simulink model "SIMULINK_PID_Tracking_R18b"  (R2018b)
settings: Solver=FixedStepAuto  StartTime=0.0  StopTime=sim_end_time  FixedStep=fixed_step_size  RelTol=1e-3
undefined symbols (not defined in the file): a, act_end, b, battery_threshold, bb, draw_gif, droneyeeUAV2_NUM, droneyeeUAV3_NUM, droneyeeUAV4_NUM, droneyeeUAV5_NUM, fixed_step_size, k, KD_x, KD_y, kd_z, KDD_x, KDD_y, KI_x, KI_y, ki_z, KII_x, KII_y, KP_x, KP_y, kp_z, KPP_x, KPP_y, lmt, omega, R, sim_end_time, uav10num, uav1num, uav2num, uav3num, uav4num, uav5num, uav6num, uav7num, uav8num, uav9num, UAV_NUM, Vel_Switch_1, Vel_Switch_10, Vel_Switch_11, Vel_Switch_12, Vel_Switch_13, Vel_Switch_14, Vel_Switch_15, Vel_Switch_16, Vel_Switch_17, Vel_Switch_18, Vel_Switch_19, Vel_Switch_2, Vel_Switch_20, Vel_Switch_3, Vel_Switch_4, Vel_Switch_5, Vel_Switch_6, Vel_Switch_7 ... (+12)
libraries: simulink x120, aerolibanimutils x1
(part 9 of 10)

== system SIMULINK_PID_Tracking_R18b/send_ctrl_signal_car1/Send Command 4/Subsystem ==
  In1 : Inport
  Compare To Constant2 : simulink/Logic and Bit Operations/Compare To Constant  relop=~=  const=0  OutDataTypeStr=boolean
  Demux : Demux  Outputs=2
  Logical Operator1 : Logic  Operator=OR  AllPortsSameDT=off  OutDataTypeStr=boolean
  Out1 : Outport
  wires:
  Demux/2 -> Logical Operator1/2
  Logical Operator1/1 -> Out1/1
  Demux/1 -> Logical Operator1/1
  Compare To Constant2/1 -> Demux/1
  In1/1 -> Compare To Constant2/1

== system SIMULINK_PID_Tracking_R18b/send_ctrl_signal_car1/Send Command 5/Subsystem ==
  In1 : Inport
  Compare To Constant2 : simulink/Logic and Bit Operations/Compare To Constant  relop=~=  const=0  OutDataTypeStr=boolean
  Demux : Demux  Outputs=2
  Logical Operator1 : Logic  Operator=OR  AllPortsSameDT=off  OutDataTypeStr=boolean
  Out1 : Outport
  wires:
  Demux/2 -> Logical Operator1/2
  Logical Operator1/1 -> Out1/1
  Demux/1 -> Logical Operator1/1
  Compare To Constant2/1 -> Demux/1
  In1/1 -> Compare To Constant2/1

== system SIMULINK_PID_Tracking_R18b/send_ctrl_signal_car1/Send Command 6/Subsystem ==
  In1 : Inport
  Compare To Constant2 : simulink/Logic and Bit Operations/Compare To Constant  relop=~=  const=0  OutDataTypeStr=boolean
  Demux : Demux  Outputs=2
  Logical Operator1 : Logic  Operator=OR  AllPortsSameDT=off  OutDataTypeStr=boolean
  Out1 : Outport
  wires:
  Demux/2 -> Logical Operator1/2
  Logical Operator1/1 -> Out1/1
  Demux/1 -> Logical Operator1/1
  Compare To Constant2/1 -> Demux/1
  In1/1 -> Compare To Constant2/1

== system SIMULINK_PID_Tracking_R18b/send_ctrl_signal_car1/Send Command 7/Subsystem ==
  In1 : Inport
  Compare To Constant2 : simulink/Logic and Bit Operations/Compare To Constant  relop=~=  const=0  OutDataTypeStr=boolean
  Demux : Demux  Outputs=2
  Logical Operator1 : Logic  Operator=OR  AllPortsSameDT=off  OutDataTypeStr=boolean
  Out1 : Outport
  wires:
  Demux/2 -> Logical Operator1/2
  Logical Operator1/1 -> Out1/1
  Demux/1 -> Logical Operator1/1
  Compare To Constant2/1 -> Demux/1
  In1/1 -> Compare To Constant2/1

== system SIMULINK_PID_Tracking_R18b/send_ctrl_signal_car1/Send Command 8/Subsystem ==
  In1 : Inport
  Compare To Constant2 : simulink/Logic and Bit Operations/Compare To Constant  relop=~=  const=0  OutDataTypeStr=boolean
  Demux : Demux  Outputs=2
  Logical Operator1 : Logic  Operator=OR  AllPortsSameDT=off  OutDataTypeStr=boolean
  Out1 : Outport
  wires:
  Demux/2 -> Logical Operator1/2
  Logical Operator1/1 -> Out1/1
  Demux/1 -> Logical Operator1/1
  Compare To Constant2/1 -> Demux/1
  In1/1 -> Compare To Constant2/1

== system SIMULINK_PID_Tracking_R18b/send_ctrl_signal_car1/Send Command 9/Subsystem ==
  In1 : Inport
  Compare To Constant2 : simulink/Logic and Bit Operations/Compare To Constant  relop=~=  const=0  OutDataTypeStr=boolean
  Demux : Demux  Outputs=2
  Logical Operator1 : Logic  Operator=OR  AllPortsSameDT=off  OutDataTypeStr=boolean
  Out1 : Outport
  wires:
  Demux/2 -> Logical Operator1/2
  Logical Operator1/1 -> Out1/1
  Demux/1 -> Logical Operator1/1
  Compare To Constant2/1 -> Demux/1
  In1/1 -> Compare To Constant2/1

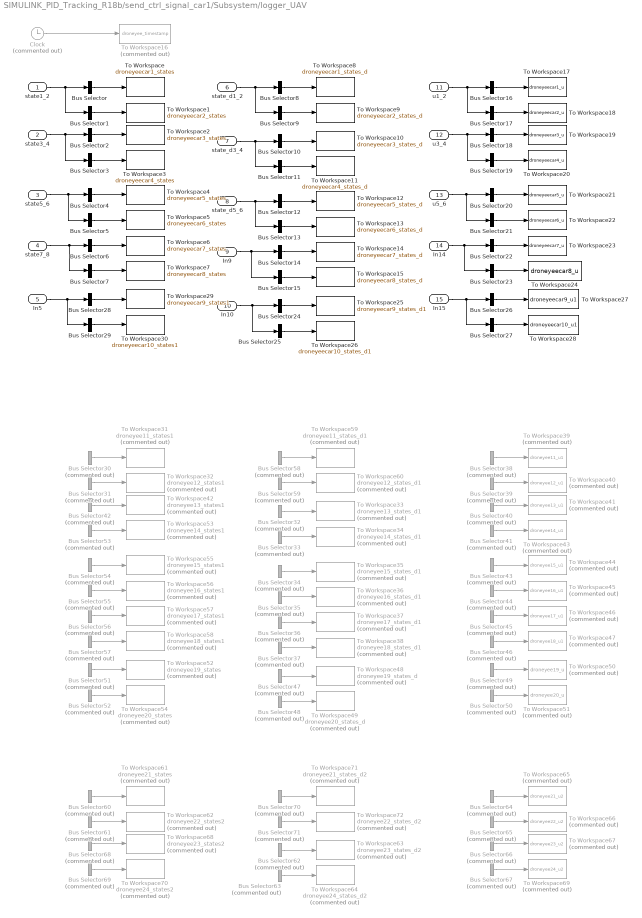
== system SIMULINK_PID_Tracking_R18b/send_ctrl_signal_car1/Subsystem/logger_UAV ==
  state1_2 : Inport
  state3_4 : Inport  Port=2
  state5_6 : Inport  Port=3
  state7_8 : Inport  Port=4
  In5 : Inport  Port=5
  state_d1_2 : Inport  Port=6
  state_d3_4 : Inport  Port=7
  state_d5_6 : Inport  Port=8
  In9 : Inport  Port=9
  In10 : Inport  Port=10
  u1_2 : Inport  Port=11
  u3_4 : Inport  Port=12
  u5_6 : Inport  Port=13
  In14 : Inport  Port=14
  In15 : Inport  Port=15
  Bus Selector : BusSelector  OutputSignals=droneyeeCAR1_states  OutputAsBus=on
  Bus Selector1 : BusSelector  OutputSignals=droneyeeCAR2_states  OutputAsBus=on
  Bus Selector10 : BusSelector  OutputSignals=droneyeeCAR3_d  OutputAsBus=on
  Bus Selector11 : BusSelector  OutputSignals=droneyeeCAR4_d  OutputAsBus=on
  Bus Selector12 : BusSelector  OutputSignals=droneyeeCAR5_d  OutputAsBus=on
  Bus Selector13 : BusSelector  OutputSignals=droneyeeCAR6_d  OutputAsBus=on
  Bus Selector14 : BusSelector  OutputSignals=droneyeeCAR7_d  OutputAsBus=on
  Bus Selector15 : BusSelector  OutputSignals=droneyeeCAR8_d  OutputAsBus=on
  Bus Selector16 : BusSelector  OutputSignals=CAR1.u_vx,CAR1.u_vy,CAR1.u_vz,CAR1.u_rate_roll,CAR1.u_rate_pitch,CAR1.u_rate_yaw  OutputAsBus=on
  Bus Selector17 : BusSelector  OutputSignals=CAR2.u_vx,CAR2.u_vy,CAR2.u_vz,CAR2.u_rate_roll,CAR2.u_rate_pitch,CAR2.u_rate_yaw  OutputAsBus=on
  Bus Selector18 : BusSelector  OutputSignals=CAR3.u_vx,CAR3.u_vy,CAR3.u_vz,CAR3.u_rate_roll,CAR3.u_rate_pitch,CAR3.u_rate_yaw  OutputAsBus=on
  Bus Selector19 : BusSelector  OutputSignals=CAR4.u_vx,CAR4.u_vy,CAR4.u_vz,CAR4.u_rate_roll,CAR4.u_rate_pitch,CAR4.u_rate_yaw  OutputAsBus=on
  Bus Selector2 : BusSelector  OutputSignals=droneyeeCAR3_states  OutputAsBus=on
  Bus Selector20 : BusSelector  OutputSignals=CAR5  OutputAsBus=on
  Bus Selector21 : BusSelector  OutputSignals=CAR6  OutputAsBus=on
  Bus Selector22 : BusSelector  OutputSignals=CAR7  OutputAsBus=on
  Bus Selector23 : BusSelector  OutputSignals=CAR8  OutputAsBus=on
  Bus Selector24 : BusSelector  OutputSignals=droneyeeCAR9_d  OutputAsBus=on
  Bus Selector25 : BusSelector  OutputSignals=droneyeeCAR10_d  OutputAsBus=on
  Bus Selector26 : BusSelector  OutputSignals=CAR9  OutputAsBus=on
  Bus Selector27 : BusSelector  OutputSignals=CAR10  OutputAsBus=on
  Bus Selector28 : BusSelector  OutputSignals=droneyeeCAR9_states  OutputAsBus=on
  Bus Selector29 : BusSelector  OutputSignals=droneyeeCAR10_states  OutputAsBus=on
  Bus Selector3 : BusSelector  OutputSignals=droneyeeCAR4_states  OutputAsBus=on
  Bus Selector30 : BusSelector  Commented=on  OutputSignals=droneyeeUAV11_states.x1,droneyeeUAV11_states.y1,droneyeeUAV11_states.z1,droneyeeUAV11_states.yaw1,droneyeeUAV11_states.vx1,droneyeeUAV11_states.vy1,droneyeeUAV11_states.vz1  OutputAsBus=on
  Bus Selector31 : BusSelector  Commented=on  OutputSignals=droneyeeUAV12_states.x2,droneyeeUAV12_states.y2,droneyeeUAV12_states.z2,droneyeeUAV12_states.yaw2,droneyeeUAV12_states.vx2,droneyeeUAV12_states.vy2,droneyeeUAV12_states.vz2  OutputAsBus=on
  Bus Selector32 : BusSelector  Commented=on  OutputSignals=droneyeeUAV13_d.x13_d,droneyeeUAV13_d.y13_d,droneyeeUAV13_d.z13_d,droneyeeUAV13_d.yaw13_d  OutputAsBus=on
  Bus Selector33 : BusSelector  Commented=on  OutputSignals=droneyeeUAV14_d.x14_d,droneyeeUAV14_d.y14_d,droneyeeUAV14_d.z14_d,droneyeeUAV14_d.yaw14_d  OutputAsBus=on
  Bus Selector34 : BusSelector  Commented=on  OutputSignals=droneyeeUAV15_d.x15_d,droneyeeUAV15_d.y15_d,droneyeeUAV15_d.z15_d,droneyeeUAV15_d.yaw15_d  OutputAsBus=on
  Bus Selector35 : BusSelector  Commented=on  OutputSignals=droneyeeUAV16_d.x16_d,droneyeeUAV16_d.y16_d,droneyeeUAV16_d.z16_d,droneyeeUAV16_d.yaw16_d  OutputAsBus=on
  Bus Selector36 : BusSelector  Commented=on  OutputSignals=droneyeeUAV17_d.x17_d,droneyeeUAV17_d.y17_d,droneyeeUAV17_d.z17_d,droneyeeUAV17_d.yaw17_d  OutputAsBus=on
  Bus Selector37 : BusSelector  Commented=on  OutputSignals=droneyeeUAV18_d.x18_d,droneyeeUAV18_d.y18_d,droneyeeUAV18_d.z18_d,droneyeeUAV18_d.yaw18_d  OutputAsBus=on
  Bus Selector38 : BusSelector  Commented=on  OutputSignals=uav1.u_vx,uav1.u_vy,uav1.u_vz,uav1.u_rate_roll,uav1.u_rate_pitch,uav1.u_rate_yaw  OutputAsBus=on
  Bus Selector39 : BusSelector  Commented=on  OutputSignals=uav2.u_vx,uav2.u_vy,uav2.u_vz,uav2.u_rate_roll,uav2.u_rate_pitch,uav2.u_rate_yaw  OutputAsBus=on
  Bus Selector4 : BusSelector  OutputSignals=droneyeeCAR5_states  OutputAsBus=on
  Bus Selector40 : BusSelector  Commented=on  OutputSignals=uav3.u_vx,uav3.u_vy,uav3.u_vz,uav3.u_rate_roll,uav3.u_rate_pitch,uav3.u_rate_yaw  OutputAsBus=on
  Bus Selector41 : BusSelector  Commented=on  OutputSignals=uav4.u_vx,uav4.u_vy,uav4.u_vz,uav4.u_rate_roll,uav4.u_rate_pitch,uav4.u_rate_yaw  OutputAsBus=on
  Bus Selector42 : BusSelector  Commented=on  OutputSignals=droneyeeUAV13_states.x3,droneyeeUAV13_states.y3,droneyeeUAV13_states.z3,droneyeeUAV13_states.yaw3,droneyeeUAV13_states.vx3,droneyeeUAV13_states.vy3,droneyeeUAV13_states.vz3  OutputAsBus=on
  Bus Selector43 : BusSelector  Commented=on  OutputSignals=uav5.u_vx,uav5.u_vy,uav5.u_vz,uav5.u_rate_roll,uav5.u_rate_pitch,uav5.u_rate_yaw  OutputAsBus=on
  Bus Selector44 : BusSelector  Commented=on  OutputSignals=uav6.u_vx,uav6.u_vy,uav6.u_vz,uav6.u_rate_roll,uav6.u_rate_pitch,uav6.u_rate_yaw  OutputAsBus=on
  Bus Selector45 : BusSelector  Commented=on  OutputSignals=uav7.u_vx,uav7.u_vy,uav7.u_vz,uav7.u_rate_roll,uav7.u_rate_pitch,uav7.u_rate_yaw  OutputAsBus=on
  Bus Selector46 : BusSelector  Commented=on  OutputSignals=uav8.u_vx,uav8.u_vy,uav8.u_vz,uav8.u_rate_roll,uav8.u_rate_pitch,uav8.u_rate_yaw  OutputAsBus=on
  Bus Selector47 : BusSelector  Commented=on  OutputSignals=droneyeeUAV19_d.x19_d,droneyeeUAV19_d.y19_d,droneyeeUAV19_d.z19_d,droneyeeUAV19_d.yaw19_d  OutputAsBus=on
  Bus Selector48 : BusSelector  Commented=on  OutputSignals=droneyeeUAV20_d.x20_d,droneyeeUAV20_d.y20_d,droneyeeUAV20_d.z20_d,droneyeeUAV20_d.yaw20_d  OutputAsBus=on
  Bus Selector49 : BusSelector  Commented=on  OutputSignals=uav9.u_vx,uav9.u_vy,uav9.u_vz,uav9.u_rate_roll,uav9.u_rate_pitch,uav9.u_rate_yaw  OutputAsBus=on
  Bus Selector5 : BusSelector  OutputSignals=droneyeeCAR6_states  OutputAsBus=on
  Bus Selector50 : BusSelector  Commented=on  OutputSignals=uav10.u_vx,uav10.u_vy,uav10.u_vz,uav10.u_rate_roll,uav10.u_rate_pitch,uav10.u_rate_yaw  OutputAsBus=on
  Bus Selector51 : BusSelector  Commented=on  OutputSignals=droneyeeUAV19_states.x9,droneyeeUAV19_states.y9,droneyeeUAV19_states.z9,droneyeeUAV19_states.yaw9,droneyeeUAV19_states.vx9,droneyeeUAV19_states.vy9,droneyeeUAV19_states.vz9  OutputAsBus=on
  Bus Selector52 : BusSelector  Commented=on  OutputSignals=droneyeeUAV20_states.x10,droneyeeUAV20_states.y10,droneyeeUAV20_states.z10,droneyeeUAV20_states.yaw10,droneyeeUAV20_states.vx10,droneyeeUAV20_states.vy10,droneyeeUAV20_states.vz10  OutputAsBus=on
  Bus Selector53 : BusSelector  Commented=on  OutputSignals=droneyeeUAV14_states.x4,droneyeeUAV14_states.y4,droneyeeUAV14_states.z4,droneyeeUAV14_states.yaw4,droneyeeUAV14_states.vx4,droneyeeUAV14_states.vy4,droneyeeUAV14_states.vz4  OutputAsBus=on
  Bus Selector54 : BusSelector  Commented=on  OutputSignals=droneyeeUAV15_states.x5,droneyeeUAV15_states.y5,droneyeeUAV15_states.z5,droneyeeUAV15_states.yaw5,droneyeeUAV15_states.vx5,droneyeeUAV15_states.vy5,droneyeeUAV15_states.vz5  OutputAsBus=on
  Bus Selector55 : BusSelector  Commented=on  OutputSignals=droneyeeUAV16_states.x6,droneyeeUAV16_states.y6,droneyeeUAV16_states.z6,droneyeeUAV16_states.yaw6,droneyeeUAV16_states.vx6,droneyeeUAV16_states.vy6,droneyeeUAV16_states.vz6  OutputAsBus=on
  Bus Selector56 : BusSelector  Commented=on  OutputSignals=droneyeeUAV17_states.x7,droneyeeUAV17_states.y7,droneyeeUAV17_states.z7,droneyeeUAV17_states.yaw7,droneyeeUAV17_states.vx7,droneyeeUAV17_states.vy7,droneyeeUAV17_states.vz7  OutputAsBus=on
  Bus Selector57 : BusSelector  Commented=on  OutputSignals=droneyeeUAV18_states.x8,droneyeeUAV18_states.y8,droneyeeUAV18_states.z8,droneyeeUAV18_states.yaw8,droneyeeUAV18_states.vx8,droneyeeUAV18_states.vy8,droneyeeUAV18_states.vz8  OutputAsBus=on
  Bus Selector58 : BusSelector  Commented=on  OutputSignals=droneyeeUAV11_d.x11_d,droneyeeUAV11_d.y11_d,droneyeeUAV11_d.z11_d,droneyeeUAV11_d.yaw11_d  OutputAsBus=on
  Bus Selector59 : BusSelector  Commented=on  OutputSignals=droneyeeUAV12_d.x12_d,droneyeeUAV12_d.y12_d,droneyeeUAV12_d.z12_d,droneyeeUAV12_d.yaw12_d  OutputAsBus=on
  Bus Selector6 : BusSelector  OutputSignals=droneyeeCAR7_states  OutputAsBus=on
  Bus Selector60 : BusSelector  Commented=on  OutputSignals=droneyeeUAV21_states.x1,droneyeeUAV21_states.y1,droneyeeUAV21_states.z1,droneyeeUAV21_states.yaw1,droneyeeUAV21_states.vx1,droneyeeUAV21_states.vy1,droneyeeUAV21_states.vz1  OutputAsBus=on
  Bus Selector61 : BusSelector  Commented=on  OutputSignals=droneyeeUAV22_states.x2,droneyeeUAV22_states.y2,droneyeeUAV22_states.z2,droneyeeUAV22_states.yaw2,droneyeeUAV22_states.vx2,droneyeeUAV22_states.vy2,droneyeeUAV22_states.vz2  OutputAsBus=on
  Bus Selector62 : BusSelector  Commented=on  OutputSignals=droneyeeUAV23_d.x23_d,droneyeeUAV23_d.y23_d,droneyeeUAV23_d.z23_d,droneyeeUAV23_d.yaw23_d  OutputAsBus=on
  Bus Selector63 : BusSelector  Commented=on  OutputSignals=droneyeeUAV24_d.x24_d,droneyeeUAV24_d.y24_d,droneyeeUAV24_d.z24_d,droneyeeUAV24_d.yaw24_d  OutputAsBus=on
  Bus Selector64 : BusSelector  Commented=on  OutputSignals=uav1.u_vx,uav1.u_vy,uav1.u_vz,uav1.u_rate_roll,uav1.u_rate_pitch,uav1.u_rate_yaw  OutputAsBus=on
  Bus Selector65 : BusSelector  Commented=on  OutputSignals=uav2.u_vx,uav2.u_vy,uav2.u_vz,uav2.u_rate_roll,uav2.u_rate_pitch,uav2.u_rate_yaw  OutputAsBus=on
  Bus Selector66 : BusSelector  Commented=on  OutputSignals=uav3.u_vx,uav3.u_vy,uav3.u_vz,uav3.u_rate_roll,uav3.u_rate_pitch,uav3.u_rate_yaw  OutputAsBus=on
  Bus Selector67 : BusSelector  Commented=on  OutputSignals=uav4.u_vx,uav4.u_vy,uav4.u_vz,uav4.u_rate_roll,uav4.u_rate_pitch,uav4.u_rate_yaw  OutputAsBus=on
  Bus Selector68 : BusSelector  Commented=on  OutputSignals=droneyeeUAV23_states.x3,droneyeeUAV23_states.y3,droneyeeUAV23_states.z3,droneyeeUAV23_states.yaw3,droneyeeUAV23_states.vx3,droneyeeUAV23_states.vy3,droneyeeUAV23_states.vz3  OutputAsBus=on
  Bus Selector69 : BusSelector  Commented=on  OutputSignals=droneyeeUAV24_states.x4,droneyeeUAV24_states.y4,droneyeeUAV24_states.z4,droneyeeUAV24_states.yaw4,droneyeeUAV24_states.vx4,droneyeeUAV24_states.vy4,droneyeeUAV24_states.vz4  OutputAsBus=on
  Bus Selector7 : BusSelector  OutputSignals=droneyeeCAR8_states  OutputAsBus=on
  Bus Selector70 : BusSelector  Commented=on  OutputSignals=droneyeeUAV21_d.x21_d,droneyeeUAV21_d.y21_d,droneyeeUAV21_d.z21_d,droneyeeUAV21_d.yaw21_d  OutputAsBus=on
  Bus Selector71 : BusSelector  Commented=on  OutputSignals=droneyeeUAV22_d.x22_d,droneyeeUAV22_d.y22_d,droneyeeUAV22_d.z22_d,droneyeeUAV22_d.yaw22_d  OutputAsBus=on
  Bus Selector8 : BusSelector  OutputSignals=droneyeeCAR1_d  OutputAsBus=on
  Bus Selector9 : BusSelector  OutputSignals=droneyeeCAR2_d  OutputAsBus=on
  Clock : Clock  Commented=on
  To Workspace : ToWorkspace  VariableName=droneyeecar1_states  SampleTime=-1
  To Workspace1 : ToWorkspace  VariableName=droneyeecar2_states  SampleTime=-1
  To Workspace10 : ToWorkspace  VariableName=droneyeecar3_states_d  SampleTime=-1
  To Workspace11 : ToWorkspace  VariableName=droneyeecar4_states_d  SampleTime=-1
  To Workspace12 : ToWorkspace  VariableName=droneyeecar5_states_d  SampleTime=-1
  To Workspace13 : ToWorkspace  VariableName=droneyeecar6_states_d  SampleTime=-1
  To Workspace14 : ToWorkspace  VariableName=droneyeecar7_states_d  SampleTime=-1
  To Workspace15 : ToWorkspace  VariableName=droneyeecar8_states_d  SampleTime=-1
  To Workspace16 : ToWorkspace  Commented=on  VariableName=droneyee_timestamp  SampleTime=-1
  To Workspace17 : ToWorkspace  VariableName=droneyeecar1_u  SampleTime=-1
  To Workspace18 : ToWorkspace  VariableName=droneyeecar2_u  SampleTime=-1
  To Workspace19 : ToWorkspace  VariableName=droneyeecar3_u  SampleTime=-1
  To Workspace2 : ToWorkspace  VariableName=droneyeecar3_states  SampleTime=-1
  To Workspace20 : ToWorkspace  VariableName=droneyeecar4_u  SampleTime=-1
  To Workspace21 : ToWorkspace  VariableName=droneyeecar5_u  SampleTime=-1
  To Workspace22 : ToWorkspace  VariableName=droneyeecar6_u  SampleTime=-1
  To Workspace23 : ToWorkspace  VariableName=droneyeecar7_u  SampleTime=-1
  To Workspace24 : ToWorkspace  VariableName=droneyeecar8_u  SampleTime=-1
  To Workspace25 : ToWorkspace  VariableName=droneyeecar9_states_d1  SampleTime=-1
  To Workspace26 : ToWorkspace  VariableName=droneyeecar10_states_d1  SampleTime=-1
  To Workspace27 : ToWorkspace  VariableName=droneyeecar9_u1  SampleTime=-1
  To Workspace28 : ToWorkspace  VariableName=droneyeecar10_u1  SampleTime=-1
  To Workspace29 : ToWorkspace  VariableName=droneyeecar9_states1  SampleTime=-1
  To Workspace3 : ToWorkspace  VariableName=droneyeecar4_states  SampleTime=-1
  To Workspace30 : ToWorkspace  VariableName=droneyeecar10_states1  SampleTime=-1
  To Workspace31 : ToWorkspace  Commented=on  VariableName=droneyee11_states1  SampleTime=-1
  To Workspace32 : ToWorkspace  Commented=on  VariableName=droneyee12_states1  SampleTime=-1
  To Workspace33 : ToWorkspace  Commented=on  VariableName=droneyee13_states_d1  SampleTime=-1
  To Workspace34 : ToWorkspace  Commented=on  VariableName=droneyee14_states_d1  SampleTime=-1
  To Workspace35 : ToWorkspace  Commented=on  VariableName=droneyee15_states_d1  SampleTime=-1
  To Workspace36 : ToWorkspace  Commented=on  VariableName=droneyee16_states_d1  SampleTime=-1
  To Workspace37 : ToWorkspace  Commented=on  VariableName=droneyee17_states_d1  SampleTime=-1
  To Workspace38 : ToWorkspace  Commented=on  VariableName=droneyee18_states_d1  SampleTime=-1
  To Workspace39 : ToWorkspace  Commented=on  VariableName=droneyee11_u1  SampleTime=-1
  To Workspace4 : ToWorkspace  VariableName=droneyeecar5_states  SampleTime=-1
  To Workspace40 : ToWorkspace  Commented=on  VariableName=droneyee12_u1  SampleTime=-1
  To Workspace41 : ToWorkspace  Commented=on  VariableName=droneyee13_u1  SampleTime=-1
  To Workspace42 : ToWorkspace  Commented=on  VariableName=droneyee13_states1  SampleTime=-1
  To Workspace43 : ToWorkspace  Commented=on  VariableName=droneyee14_u1  SampleTime=-1
  To Workspace44 : ToWorkspace  Commented=on  VariableName=droneyee15_u1  SampleTime=-1
  To Workspace45 : ToWorkspace  Commented=on  VariableName=droneyee16_u1  SampleTime=-1
  To Workspace46 : ToWorkspace  Commented=on  VariableName=droneyee17_u1  SampleTime=-1
  To Workspace47 : ToWorkspace  Commented=on  VariableName=droneyee18_u1  SampleTime=-1
  To Workspace48 : ToWorkspace  Commented=on  VariableName=droneyee19_states_d  SampleTime=-1
  To Workspace49 : ToWorkspace  Commented=on  VariableName=droneyee20_states_d  SampleTime=-1
  To Workspace5 : ToWorkspace  VariableName=droneyeecar6_states  SampleTime=-1
  To Workspace50 : ToWorkspace  Commented=on  VariableName=droneyee19_u  SampleTime=-1
  To Workspace51 : ToWorkspace  Commented=on  VariableName=droneyee20_u  SampleTime=-1
  To Workspace52 : ToWorkspace  Commented=on  VariableName=droneyee19_states  SampleTime=-1
  To Workspace53 : ToWorkspace  Commented=on  VariableName=droneyee14_states1  SampleTime=-1
  To Workspace54 : ToWorkspace  Commented=on  VariableName=droneyee20_states  SampleTime=-1
  To Workspace55 : ToWorkspace  Commented=on  VariableName=droneyee15_states1  SampleTime=-1
  To Workspace56 : ToWorkspace  Commented=on  VariableName=droneyee16_states1  SampleTime=-1
  To Workspace57 : ToWorkspace  Commented=on  VariableName=droneyee17_states1  SampleTime=-1
  To Workspace58 : ToWorkspace  Commented=on  VariableName=droneyee18_states1  SampleTime=-1
  To Workspace59 : ToWorkspace  Commented=on  VariableName=droneyee11_states_d1  SampleTime=-1
  To Workspace6 : ToWorkspace  VariableName=droneyeecar7_states  SampleTime=-1
  To Workspace60 : ToWorkspace  Commented=on  VariableName=droneyee12_states_d1  SampleTime=-1
  To Workspace61 : ToWorkspace  Commented=on  VariableName=droneyee21_states  SampleTime=-1
  To Workspace62 : ToWorkspace  Commented=on  VariableName=droneyee22_states2  SampleTime=-1
  To Workspace63 : ToWorkspace  Commented=on  VariableName=droneyee23_states_d2  SampleTime=-1
  To Workspace64 : ToWorkspace  Commented=on  VariableName=droneyee24_states_d2  SampleTime=-1
  To Workspace65 : ToWorkspace  Commented=on  VariableName=droneyee21_u2  SampleTime=-1
  To Workspace66 : ToWorkspace  Commented=on  VariableName=droneyee22_u2  SampleTime=-1
  To Workspace67 : ToWorkspace  Commented=on  VariableName=droneyee23_u2  SampleTime=-1
  To Workspace68 : ToWorkspace  Commented=on  VariableName=droneyee23_states2  SampleTime=-1
  To Workspace69 : ToWorkspace  Commented=on  VariableName=droneyee24_u2  SampleTime=-1
  To Workspace7 : ToWorkspace  VariableName=droneyeecar8_states  SampleTime=-1
  To Workspace70 : ToWorkspace  Commented=on  VariableName=droneyee24_states2  SampleTime=-1
  To Workspace71 : ToWorkspace  Commented=on  VariableName=droneyee21_states_d2  SampleTime=-1
  To Workspace72 : ToWorkspace  Commented=on  VariableName=droneyee22_states_d2  SampleTime=-1
  To Workspace8 : ToWorkspace  VariableName=droneyeecar1_states_d  SampleTime=-1
  To Workspace9 : ToWorkspace  VariableName=droneyeecar2_states_d  SampleTime=-1
  wires:
  state1_2/1 -> Bus Selector1/1, Bus Selector/1
  Bus Selector/1 -> To Workspace/1
  Bus Selector1/1 -> To Workspace1/1
  Bus Selector3/1 -> To Workspace3/1
  Bus Selector2/1 -> To Workspace2/1
  state3_4/1 -> Bus Selector3/1, Bus Selector2/1
  Bus Selector5/1 -> To Workspace5/1
  Bus Selector4/1 -> To Workspace4/1
  Bus Selector7/1 -> To Workspace7/1
  Bus Selector6/1 -> To Workspace6/1
  Bus Selector9/1 -> To Workspace9/1
  Bus Selector8/1 -> To Workspace8/1
  state_d1_2/1 -> Bus Selector9/1, Bus Selector8/1
  Bus Selector10/1 -> To Workspace10/1
  Bus Selector11/1 -> To Workspace11/1
  Bus Selector12/1 -> To Workspace12/1
  state_d3_4/1 -> Bus Selector11/1, Bus Selector10/1
  state_d5_6/1 -> Bus Selector13/1, Bus Selector12/1
  Bus Selector15/1 -> To Workspace15/1
  Bus Selector13/1 -> To Workspace13/1
  Bus Selector14/1 -> To Workspace14/1
  Clock/1 -> To Workspace16/1
  Bus Selector18/1 -> To Workspace19/1
  Bus Selector19/1 -> To Workspace20/1
  Bus Selector20/1 -> To Workspace21/1
  u5_6/1 -> Bus Selector21/1, Bus Selector20/1
  Bus Selector21/1 -> To Workspace22/1
  Bus Selector23/1 -> To Workspace24/1
  u1_2/1 -> Bus Selector17/1, Bus Selector16/1
  Bus Selector17/1 -> To Workspace18/1
  Bus Selector16/1 -> To Workspace17/1
  u3_4/1 -> Bus Selector19/1, Bus Selector18/1
  Bus Selector22/1 -> To Workspace23/1
  Bus Selector27/1 -> To Workspace28/1
  Bus Selector26/1 -> To Workspace27/1
  Bus Selector29/1 -> To Workspace30/1
  Bus Selector25/1 -> To Workspace26/1
  Bus Selector28/1 -> To Workspace29/1
  Bus Selector24/1 -> To Workspace25/1
  Bus Selector40/1 -> To Workspace41/1
  Bus Selector36/1 -> To Workspace37/1
  Bus Selector55/1 -> To Workspace56/1
  Bus Selector43/1 -> To Workspace44/1
  Bus Selector48/1 -> To Workspace49/1
  Bus Selector52/1 -> To Workspace54/1
  Bus Selector34/1 -> To Workspace35/1
  Bus Selector39/1 -> To Workspace40/1
  Bus Selector35/1 -> To Workspace36/1
  Bus Selector47/1 -> To Workspace48/1
  Bus Selector54/1 -> To Workspace55/1
  Bus Selector37/1 -> To Workspace38/1
  Bus Selector42/1 -> To Workspace42/1
  Bus Selector56/1 -> To Workspace57/1
  Bus Selector58/1 -> To Workspace59/1
  Bus Selector32/1 -> To Workspace33/1
  Bus Selector57/1 -> To Workspace58/1
  Bus Selector30/1 -> To Workspace31/1
  Bus Selector45/1 -> To Workspace46/1
  Bus Selector31/1 -> To Workspace32/1
  Bus Selector33/1 -> To Workspace34/1
  Bus Selector59/1 -> To Workspace60/1
  Bus Selector44/1 -> To Workspace45/1
  Bus Selector46/1 -> To Workspace47/1
  Bus Selector51/1 -> To Workspace52/1
  Bus Selector53/1 -> To Workspace53/1
  Bus Selector38/1 -> To Workspace39/1
  Bus Selector50/1 -> To Workspace51/1
  Bus Selector49/1 -> To Workspace50/1
  Bus Selector41/1 -> To Workspace43/1
  Bus Selector68/1 -> To Workspace68/1
  Bus Selector67/1 -> To Workspace69/1
  Bus Selector69/1 -> To Workspace70/1
  Bus Selector71/1 -> To Workspace72/1
  Bus Selector66/1 -> To Workspace67/1
  Bus Selector62/1 -> To Workspace63/1
  Bus Selector61/1 -> To Workspace62/1
  Bus Selector63/1 -> To Workspace64/1
  Bus Selector65/1 -> To Workspace66/1
  Bus Selector60/1 -> To Workspace61/1
  Bus Selector64/1 -> To Workspace65/1
  Bus Selector70/1 -> To Workspace71/1
  state7_8/1 -> Bus Selector7/1, Bus Selector6/1
  state5_6/1 -> Bus Selector5/1, Bus Selector4/1
  In9/1 -> Bus Selector15/1, Bus Selector14/1
  In5/1 -> Bus Selector29/1, Bus Selector28/1
  In10/1 -> Bus Selector25/1, Bus Selector24/1
  In14/1 -> Bus Selector23/1, Bus Selector22/1
  In15/1 -> Bus Selector27/1, Bus Selector26/1

== matlab function SIMULINK_PID_Tracking_R18b/control system_UAV/Baseline Controller2/MATLAB Function ==
  data: u input; y output; a input
function y = fcn(u,a)
y = satgd(u,a);

== matlab function SIMULINK_PID_Tracking_R18b/CMD_UAV/CMD2/MATLAB Function1 ==
  settings: updateMethod=DISCRETE
  data: x_d input; y_d input; z_d input; timestamp input; x input; y input; z input; battery_status input; sim_time_end input; x_d_ output; battery_threshold input; z_d_for_land input; y_d_ output; z_d_ output; UAV_NUM input
function [x_d_, y_d_, z_d_] = fcn(x_d, y_d, z_d, timestamp, x,y,z,battery_status, sim_time_end,battery_threshold, z_d_for_land, UAV_NUM)
persistent s_x s_y s_z ready_land
if isempty(s_x)
    s_x = x;
end
if isempty(s_y)
    s_y = y;
end
if isempty(s_z)
    s_z = z;
end
if isempty(ready_land)
    ready_land = false;
end
    
battery_low = false;
for i = 1:UAV_NUM
    if battery_status(i) < battery_threshold
        battery_low = true;
        break;
    end
end
if sim_time_end - timestamp < 1
    tello_stop = true;
else
    tello_stop = false;
end
if battery_low || tello_stop
    if ~ready_land
        ready_land = true;
    end
    z_d_ = z_d_for_land;
    x_d_ = s_x;
    y_d_ = s_y;
else
   ready_land = false;
   s_x = x;
   s_y = y;
   x_d_ = x_d;
   y_d_ = y_d;
   z_d_ = z_d;
end

== matlab function SIMULINK_PID_Tracking_R18b/CMD_UAV/CMD2/Subsystem/MATLAB Function ==
  settings: updateMethod=DISCRETE
  data: timestamp input; uavnum input; x_ output; y_ output; z_ output; switch_flag input; stas input; trj_flag input; form_flag input; avo_flag input
function [x_, y_, z_] = fcn(timestamp, uavnum,switch_flag,stas,trj_flag,form_flag,avo_flag)

[x_,y_,z_]=trjuav(timestamp,uavnum,switch_flag,stas,trj_flag,form_flag,avo_flag);

== matlab function SIMULINK_PID_Tracking_R18b/CMD_UAV/CMD1/Subsystem/MATLAB Function ==
  settings: updateMethod=DISCRETE
  data: timestamp input; uavnum input; x_ output; y_ output; z_ output; switch_flag input; stas input; trj_flag input; form_flag input; avo_flag input; ref input
function [x_, y_, z_] = fcn(timestamp, uavnum,switch_flag,stas,trj_flag,form_flag,avo_flag,ref)

% [x_,y_,z_]=trjuav(timestamp,uavnum,switch_flag,stas,trj_flag,form_flag,avo_flag);
[x_,y_,z_]=trjuav_DMP(timestamp,uavnum,switch_flag,stas,trj_flag,form_flag,avo_flag,ref);

== matlab function SIMULINK_PID_Tracking_R18b/CMD_UAV/CMD4/MATLAB Function1 ==
  settings: updateMethod=DISCRETE
  data: x_d input; y_d input; z_d input; timestamp input; x input; y input; z input; battery_status input; sim_time_end input; x_d_ output; battery_threshold input; z_d_for_land input; y_d_ output; z_d_ output; UAV_NUM input
function [x_d_, y_d_, z_d_] = fcn(x_d, y_d, z_d, timestamp, x,y,z,battery_status, sim_time_end,battery_threshold, z_d_for_land, UAV_NUM)
persistent s_x s_y s_z ready_land
if isempty(s_x)
    s_x = x;
end
if isempty(s_y)
    s_y = y;
end
if isempty(s_z)
    s_z = z;
end
if isempty(ready_land)
    ready_land = false;
end
    
battery_low = false;
for i = 1:UAV_NUM
    if battery_status(i) < battery_threshold
        battery_low = true;
        break;
    end
end
if sim_time_end - timestamp < 1
    tello_stop = true;
else
    tello_stop = false;
end
if battery_low || tello_stop
    if ~ready_land
        ready_land = true;
    end
    z_d_ = z_d_for_land;
    x_d_ = s_x;
    y_d_ = s_y;
else
   ready_land = false;
   s_x = x;
   s_y = y;
   x_d_ = x_d;
   y_d_ = y_d;
   z_d_ = z_d;
end

== matlab function SIMULINK_PID_Tracking_R18b/CMD_UAV/CMD4/Subsystem/MATLAB Function ==
  settings: updateMethod=DISCRETE
  data: timestamp input; uavnum input; x_ output; y_ output; z_ output; switch_flag input; stas input; trj_flag input; form_flag input; avo_flag input
function [x_, y_, z_] = fcn(timestamp, uavnum,switch_flag,stas,trj_flag,form_flag,avo_flag)

[x_,y_,z_]=trjuav(timestamp,uavnum,switch_flag,stas,trj_flag,form_flag,avo_flag);

== matlab function SIMULINK_PID_Tracking_R18b/plot/MATLAB Function ==
  data: x1 input; y1 input; z1 input; x2 input; y2 input; z2 input; x3 input; y3 input; z3 input; x4 input; y4 input; z4 input; x5 input; y5 input; z5 input; x6 input; y6 input; z6 input; x7 input; y7 input; z7 input; x8 input; y8 input; z8 input; x9 input; y9 input; z9 input; x10 input; y10 input; z10 input; x11 input; y11 input; z11 input; x12 input; y12 input; z12 input; x13 input; y13 input; z13 input; x14 input; y14 input; z14 input; x15 input; y15 input; z15 input; x16 input; y16 input; z16 input; x17 input; y17 input; z17 input; x18 input; y18 input; z18 input; x19 input; y19 input; z19 input; x20 input; y20 input; z20 input; x21 input; y21 input; z21 input; x22 input; y22 input; z22 input; x23 input; y23 input; z23 input; x24 input; y24 input; z24 input; time_step input; act_end input; XMIN input; XMAX input; YMIN input; YMAX input; ZMIN input; ZMAX input; a input; b input; k input; bb input; w1 input; w2 input; draw_gif input
function f_eight_shaped(x1, y1, z1, x2, y2, z2, x3, y3, z3,x4, y4, z4, x5, y5, z5, x6, y6, z6, x7, y7, z7,x8, y8, z8,x9, y9, z9,x10,y10,z10,x11, y11, z11, x12, y12, z12, x13, y13, z13,x14, y14, z14, x15, y15, z15, x16, y16, z16, x17, y17, z17,x18, y18, z18,x19, y19, z19,x20,y20,z20,x21, y21, z21, x22, y22, z22, x23, y23, z23,x24, y24, z24,time_step, act_end, XMIN,XMAX, YMIN, YMAX, ZMIN, ZMAX, a, b, k, bb, w1, w2,draw_gif)

% persistent index
% if isempty(index)
%     index = 0;
% end
% length = 8000;
% persistent posd_x  posd_y posd_z
% if isempty(posd_x)
%     posd_x = zeros(length,1);
% end
% if isempty(posd_y)
%     posd_y = zeros(length,1);
% end
% if isempty(posd_z)
%     posd_z = zeros(length,1);
% end
% 
% index = index + 1;
% if index <= 1
%     axis([XMIN*1.2 XMAX*1.2 YMIN*1.2 YMAX*1.2 ZMIN*0.5 ZMAX*1.2]);
%     xlabel('X(m)');
%     ylabel('Y(m)');
%     zlabel('Z(m)');
%     box on;
%     i= 0;
%     for t = 0:time_step:act_end
%         i = i+1;
%         posd_x(i) = a*cos(w1*t);
%         posd_y(i) = b*sin(w2*t);
%         posd_z(i) = k*posd_x(i) + bb;
%     end
% else
    cla;
    hold on
    %data_num = floor(act_end/time_step);
%     plot3(posd_x(1:data_num), posd_y(1:data_num), posd_z(1:data_num));
    plot3(x1,y1,z1,'ro');
    plot3(x2,y2,z2,'g*');
    plot3(x3,y3,z3,'bo');
    plot3(x4,y4,z4,'y*');
    plot3(x5,y5,z5,'co');
    plot3(x6,y6,z6,'m*');
    plot3(x7,y7,z7,'ko');
    plot3(x8,y8,z8,'r*');
    plot3(x9,y9,z9,'cp');
    plot3(x10,y10,z10,'bs');
%     coder.extrinsic('getframe')
%     if draw_gif
%          frame=getframe(gcf);
%          imind=frame2im(frame);
%          [imind,cm] = rgb2ind(imind,256);
%          if index <=2
%              imwrite(imind,cm,'eight-shaped.gif','gif', 'Loopcount',inf,'DelayTime',time_step);
%          else
%              imwrite(imind,cm,'eight-shaped.gif','gif','WriteMode','append','DelayTime',time_step);
%          end
%     end
end

== matlab function SIMULINK_PID_Tracking_R18b/CMD_UAV/CMD5/MATLAB Function1 ==
  settings: updateMethod=DISCRETE
  data: x_d input; y_d input; z_d input; timestamp input; x input; y input; z input; battery_status input; sim_time_end input; x_d_ output; battery_threshold input; z_d_for_land input; y_d_ output; z_d_ output; UAV_NUM input
function [x_d_, y_d_, z_d_] = fcn(x_d, y_d, z_d, timestamp, x,y,z,battery_status, sim_time_end,battery_threshold, z_d_for_land, UAV_NUM)
persistent s_x s_y s_z ready_land
if isempty(s_x)
    s_x = x;
end
if isempty(s_y)
    s_y = y;
end
if isempty(s_z)
    s_z = z;
end
if isempty(ready_land)
    ready_land = false;
end
    
battery_low = false;
for i = 1:UAV_NUM
    if battery_status(i) < battery_threshold
        battery_low = true;
        break;
    end
end
if sim_time_end - timestamp < 1
    tello_stop = true;
else
    tello_stop = false;
end
if battery_low || tello_stop
    if ~ready_land
        ready_land = true;
    end
    z_d_ = z_d_for_land;
    x_d_ = s_x;
    y_d_ = s_y;
else
   ready_land = false;
   s_x = x;
   s_y = y;
   x_d_ = x_d;
   y_d_ = y_d;
   z_d_ = z_d;
end

== matlab function SIMULINK_PID_Tracking_R18b/CMD_UAV/CMD5/Subsystem/MATLAB Function ==
  settings: updateMethod=DISCRETE
  data: timestamp input; uavnum input; x_ output; y_ output; z_ output; switch_flag input; stas input; trj_flag input; form_flag input; avo_flag input
function [x_, y_, z_] = fcn(timestamp, uavnum,switch_flag,stas,trj_flag,form_flag,avo_flag)

[x_,y_,z_]=trjuav(timestamp,uavnum,switch_flag,stas,trj_flag,form_flag,avo_flag);

== matlab function SIMULINK_PID_Tracking_R18b/CMD_UAV/CMD3/Subsystem/MATLAB Function ==
  settings: updateMethod=DISCRETE
  data: timestamp input; uavnum input; x_ output; y_ output; z_ output; switch_flag input; stas input; trj_flag input; form_flag input; avo_flag input; ref input
% function [x_, y_, z_] = fcn(timestamp, uavnum,switch_flag,stas,trj_flag,form_flag,avo_flag)
% 
% [x_,y_,z_]=trjuav(timestamp,uavnum,switch_flag,stas,trj_flag,form_flag,avo_flag);
function [x_, y_, z_] = fcn(timestamp, uavnum,switch_flag,stas,trj_flag,form_flag,avo_flag,ref)

% [x_,y_,z_]=trjuav(timestamp,uavnum,switch_flag,stas,trj_flag,form_flag,avo_flag);
[x_,y_,z_]=trjuav_DMP(timestamp,uavnum,switch_flag,stas,trj_flag,form_flag,avo_flag,ref);

== matlab function SIMULINK_PID_Tracking_R18b/CMD_car1/CMD1/MATLAB Function1 ==
  settings: updateMethod=DISCRETE
  data: x_d input; y_d input; z_d input; timestamp input; x input; y input; z input; battery_status input; sim_time_end input; x_d_ output; battery_threshold input; z_d_for_land input; y_d_ output; z_d_ output; UAV_NUM input
function [x_d_, y_d_, z_d_] = fcn(x_d, y_d, z_d, timestamp, x,y,z,battery_status, sim_time_end,battery_threshold, z_d_for_land, UAV_NUM)
persistent s_x s_y s_z ready_land
if isempty(s_x)
    s_x = x;
end
if isempty(s_y)
    s_y = y;
end
if isempty(s_z)
    s_z = z;
end
if isempty(ready_land)
    ready_land = false;
end
    
battery_low = false;
for i = 1:UAV_NUM
    if battery_status(i) < battery_threshold
        battery_low = true;
        break;
    end
end
if sim_time_end - timestamp < 1
    tello_stop = true;
else
    tello_stop = false;
end
if battery_low || tello_stop
    if ~ready_land
        ready_land = true;
    end
    z_d_ = z_d_for_land;
    x_d_ = s_x;
    y_d_ = s_y;
else
   ready_land = false;
   s_x = x;
   s_y = y;
   x_d_ = x_d;
   y_d_ = y_d;
   z_d_ = z_d;
end

== matlab function SIMULINK_PID_Tracking_R18b/control system_UAV/Baseline Controller1/MATLAB Function ==
  data: u input; y output; a input
function y = fcn(u,a)
y = satgd(u,a);

== matlab function SIMULINK_PID_Tracking_R18b/CMD_UAV/CMD3/MATLAB Function1 ==
  settings: updateMethod=DISCRETE
  data: x_d input; y_d input; z_d input; timestamp input; x input; y input; z input; battery_status input; sim_time_end input; x_d_ output; battery_threshold input; z_d_for_land input; y_d_ output; z_d_ output; UAV_NUM input
function [x_d_, y_d_, z_d_] = fcn(x_d, y_d, z_d, timestamp, x,y,z,battery_status, sim_time_end,battery_threshold, z_d_for_land, UAV_NUM)
persistent s_x s_y s_z ready_land
if isempty(s_x)
    s_x = x;
end
if isempty(s_y)
    s_y = y;
end
if isempty(s_z)
    s_z = z;
end
if isempty(ready_land)
    ready_land = false;
end
    
battery_low = false;
for i = 1:UAV_NUM
    if battery_status(i) < battery_threshold
        battery_low = true;
        break;
    end
end
if sim_time_end - timestamp < 1
    tello_stop = true;
else
    tello_stop = false;
end
if battery_low || tello_stop
    if ~ready_land
        ready_land = true;
    end
    z_d_ = z_d_for_land;
    x_d_ = s_x;
    y_d_ = s_y;
else
   ready_land = false;
   s_x = x;
   s_y = y;
   x_d_ = x_d;
   y_d_ = y_d;
   z_d_ = z_d;
end

== matlab function SIMULINK_PID_Tracking_R18b/CMD_car1/CMD1/Subsystem/MATLAB Function ==
  settings: updateMethod=DISCRETE
  data: timestamp input; uavnum input; x_ output; y_ output; z_ output; switch_flag input; stas input; trj_flag input; form_flag input; avo_flag input
function [x_, y_, z_] = fcn(timestamp, uavnum,switch_flag,stas,trj_flag,form_flag,avo_flag)

[x_,y_,z_]=trjcar(timestamp,uavnum,switch_flag,stas,trj_flag,form_flag,avo_flag);

== matlab function SIMULINK_PID_Tracking_R18b/CMD_car1/CMD10/MATLAB Function1 ==
  settings: updateMethod=DISCRETE
  data: x_d input; y_d input; z_d input; timestamp input; x input; y input; z input; battery_status input; sim_time_end input; x_d_ output; battery_threshold input; z_d_for_land input; y_d_ output; z_d_ output; UAV_NUM input
function [x_d_, y_d_, z_d_] = fcn(x_d, y_d, z_d, timestamp, x,y,z,battery_status, sim_time_end,battery_threshold, z_d_for_land, UAV_NUM)
persistent s_x s_y s_z ready_land
if isempty(s_x)
    s_x = x;
end
if isempty(s_y)
    s_y = y;
end
if isempty(s_z)
    s_z = z;
end
if isempty(ready_land)
    ready_land = false;
end
    
battery_low = false;
for i = 1:UAV_NUM
    if battery_status(i) < battery_threshold
        battery_low = true;
        break;
    end
end
if sim_time_end - timestamp < 1
    tello_stop = true;
else
    tello_stop = false;
end
if battery_low || tello_stop
    if ~ready_land
        ready_land = true;
    end
    z_d_ = z_d_for_land;
    x_d_ = s_x;
    y_d_ = s_y;
else
   ready_land = false;
   s_x = x;
   s_y = y;
   x_d_ = x_d;
   y_d_ = y_d;
   z_d_ = z_d;
end

== matlab function SIMULINK_PID_Tracking_R18b/CMD_UAV/CMD1/MATLAB Function1 ==
  settings: updateMethod=DISCRETE
  data: x_d input; y_d input; z_d input; timestamp input; x input; y input; z input; battery_status input; sim_time_end input; x_d_ output; battery_threshold input; z_d_for_land input; y_d_ output; z_d_ output; UAV_NUM input
function [x_d_, y_d_, z_d_] = fcn(x_d, y_d, z_d, timestamp, x,y,z,battery_status, sim_time_end,battery_threshold, z_d_for_land, UAV_NUM)
persistent s_x s_y s_z ready_land
if isempty(s_x)
    s_x = x;
end
if isempty(s_y)
    s_y = y;
end
if isempty(s_z)
    s_z = z;
end
if isempty(ready_land)
    ready_land = false;
end
    
battery_low = false;
for i = 1:UAV_NUM
    if battery_status(i) < battery_threshold
        battery_low = true;
        break;
    end
end
if sim_time_end - timestamp < 1
    tello_stop = true;
else
    tello_stop = false;
end
if battery_low || tello_stop
    if ~ready_land
        ready_land = true;
    end
    z_d_ = z_d_for_land;
    x_d_ = s_x;
    y_d_ = s_y;
else
   ready_land = false;
   s_x = x;
   s_y = y;
   x_d_ = x_d;
   y_d_ = y_d;
   z_d_ = z_d;
end

== matlab function SIMULINK_PID_Tracking_R18b/CMD_car1/CMD10/Subsystem/MATLAB Function ==
  settings: updateMethod=DISCRETE
  data: timestamp input; uavnum input; x_ output; y_ output; z_ output; switch_flag input; stas input; trj_flag input; form_flag input; avo_flag input
function [x_, y_, z_] = fcn(timestamp, uavnum,switch_flag,stas,trj_flag,form_flag,avo_flag)

[x_,y_,z_]=trjcar(timestamp,uavnum,switch_flag,stas,trj_flag,form_flag,avo_flag);

== matlab function SIMULINK_PID_Tracking_R18b/CMD_car1/CMD2/MATLAB Function1 ==
  settings: updateMethod=DISCRETE
  data: x_d input; y_d input; z_d input; timestamp input; x input; y input; z input; battery_status input; sim_time_end input; x_d_ output; battery_threshold input; z_d_for_land input; y_d_ output; z_d_ output; UAV_NUM input
function [x_d_, y_d_, z_d_] = fcn(x_d, y_d, z_d, timestamp, x,y,z,battery_status, sim_time_end,battery_threshold, z_d_for_land, UAV_NUM)
persistent s_x s_y s_z ready_land
if isempty(s_x)
    s_x = x;
end
if isempty(s_y)
    s_y = y;
end
if isempty(s_z)
    s_z = z;
end
if isempty(ready_land)
    ready_land = false;
end
    
battery_low = false;
for i = 1:UAV_NUM
    if battery_status(i) < battery_threshold
        battery_low = true;
        break;
    end
end
if sim_time_end - timestamp < 1
    tello_stop = true;
else
    tello_stop = false;
end
if battery_low || tello_stop
    if ~ready_land
        ready_land = true;
    end
    z_d_ = z_d_for_land;
    x_d_ = s_x;
    y_d_ = s_y;
else
   ready_land = false;
   s_x = x;
   s_y = y;
   x_d_ = x_d;
   y_d_ = y_d;
   z_d_ = z_d;
end

== matlab function SIMULINK_PID_Tracking_R18b/CMD_car1/CMD2/Subsystem/MATLAB Function ==
  settings: updateMethod=DISCRETE
  data: timestamp input; uavnum input; x_ output; y_ output; z_ output; switch_flag input; stas input; trj_flag input; form_flag input; avo_flag input
function [x_, y_, z_] = fcn(timestamp, uavnum,switch_flag,stas,trj_flag,form_flag,avo_flag)

[x_,y_,z_]=trjcar(timestamp,uavnum,switch_flag,stas,trj_flag,form_flag,avo_flag);

== matlab function SIMULINK_PID_Tracking_R18b/CMD_car1/CMD3/MATLAB Function1 ==
  settings: updateMethod=DISCRETE
  data: x_d input; y_d input; z_d input; timestamp input; x input; y input; z input; battery_status input; sim_time_end input; x_d_ output; battery_threshold input; z_d_for_land input; y_d_ output; z_d_ output; UAV_NUM input
function [x_d_, y_d_, z_d_] = fcn(x_d, y_d, z_d, timestamp, x,y,z,battery_status, sim_time_end,battery_threshold, z_d_for_land, UAV_NUM)
persistent s_x s_y s_z ready_land
if isempty(s_x)
    s_x = x;
end
if isempty(s_y)
    s_y = y;
end
if isempty(s_z)
    s_z = z;
end
if isempty(ready_land)
    ready_land = false;
end
    
battery_low = false;
for i = 1:UAV_NUM
    if battery_status(i) < battery_threshold
        battery_low = true;
        break;
    end
end
if sim_time_end - timestamp < 1
    tello_stop = true;
else
    tello_stop = false;
end
if battery_low || tello_stop
    if ~ready_land
        ready_land = true;
    end
    z_d_ = z_d_for_land;
    x_d_ = s_x;
    y_d_ = s_y;
else
   ready_land = false;
   s_x = x;
   s_y = y;
   x_d_ = x_d;
   y_d_ = y_d;
   z_d_ = z_d;
end

== matlab function SIMULINK_PID_Tracking_R18b/CMD_car1/CMD3/Subsystem/MATLAB Function ==
  settings: updateMethod=DISCRETE
  data: timestamp input; uavnum input; x_ output; y_ output; z_ output; switch_flag input; stas input; trj_flag input; form_flag input; avo_flag input
function [x_, y_, z_] = fcn(timestamp, uavnum,switch_flag,stas,trj_flag,form_flag,avo_flag)

[x_,y_,z_]=trjcar(timestamp,uavnum,switch_flag,stas,trj_flag,form_flag,avo_flag);

== matlab function SIMULINK_PID_Tracking_R18b/CMD_UAV/CMD6/MATLAB Function1 ==
  settings: updateMethod=DISCRETE
  data: x_d input; y_d input; z_d input; timestamp input; x input; y input; z input; battery_status input; sim_time_end input; x_d_ output; battery_threshold input; z_d_for_land input; y_d_ output; z_d_ output; UAV_NUM input
function [x_d_, y_d_, z_d_] = fcn(x_d, y_d, z_d, timestamp, x,y,z,battery_status, sim_time_end,battery_threshold, z_d_for_land, UAV_NUM)
persistent s_x s_y s_z ready_land
if isempty(s_x)
    s_x = x;
end
if isempty(s_y)
    s_y = y;
end
if isempty(s_z)
    s_z = z;
end
if isempty(ready_land)
    ready_land = false;
end
    
battery_low = false;
for i = 1:UAV_NUM
    if battery_status(i) < battery_threshold
        battery_low = true;
        break;
    end
end
if sim_time_end - timestamp < 1
    tello_stop = true;
else
    tello_stop = false;
end
if battery_low || tello_stop
    if ~ready_land
        ready_land = true;
    end
    z_d_ = z_d_for_land;
    x_d_ = s_x;
    y_d_ = s_y;
else
   ready_land = false;
   s_x = x;
   s_y = y;
   x_d_ = x_d;
   y_d_ = y_d;
   z_d_ = z_d;
end

== matlab function SIMULINK_PID_Tracking_R18b/CMD_car1/CMD4/MATLAB Function1 ==
  settings: updateMethod=DISCRETE
  data: x_d input; y_d input; z_d input; timestamp input; x input; y input; z input; battery_status input; sim_time_end input; x_d_ output; battery_threshold input; z_d_for_land input; y_d_ output; z_d_ output; UAV_NUM input
function [x_d_, y_d_, z_d_] = fcn(x_d, y_d, z_d, timestamp, x,y,z,battery_status, sim_time_end,battery_threshold, z_d_for_land, UAV_NUM)
persistent s_x s_y s_z ready_land
if isempty(s_x)
    s_x = x;
end
if isempty(s_y)
    s_y = y;
end
if isempty(s_z)
    s_z = z;
end
if isempty(ready_land)
    ready_land = false;
end
    
battery_low = false;
for i = 1:UAV_NUM
    if battery_status(i) < battery_threshold
        battery_low = true;
        break;
    end
end
if sim_time_end - timestamp < 1
    tello_stop = true;
else
    tello_stop = false;
end
if battery_low || tello_stop
    if ~ready_land
        ready_land = true;
    end
    z_d_ = z_d_for_land;
    x_d_ = s_x;
    y_d_ = s_y;
else
   ready_land = false;
   s_x = x;
   s_y = y;
   x_d_ = x_d;
   y_d_ = y_d;
   z_d_ = z_d;
end

== matlab function SIMULINK_PID_Tracking_R18b/CMD_car1/CMD4/Subsystem/MATLAB Function ==
  settings: updateMethod=DISCRETE
  data: timestamp input; uavnum input; x_ output; y_ output; z_ output; switch_flag input; stas input; trj_flag input; form_flag input; avo_flag input
function [x_, y_, z_] = fcn(timestamp, uavnum,switch_flag,stas,trj_flag,form_flag,avo_flag)

[x_,y_,z_]=trjcar(timestamp,uavnum,switch_flag,stas,trj_flag,form_flag,avo_flag);

== matlab function SIMULINK_PID_Tracking_R18b/CMD_car1/CMD5/MATLAB Function1 ==
  settings: updateMethod=DISCRETE
  data: x_d input; y_d input; z_d input; timestamp input; x input; y input; z input; battery_status input; sim_time_end input; x_d_ output; battery_threshold input; z_d_for_land input; y_d_ output; z_d_ output; UAV_NUM input
function [x_d_, y_d_, z_d_] = fcn(x_d, y_d, z_d, timestamp, x,y,z,battery_status, sim_time_end,battery_threshold, z_d_for_land, UAV_NUM)
persistent s_x s_y s_z ready_land
if isempty(s_x)
    s_x = x;
end
if isempty(s_y)
    s_y = y;
end
if isempty(s_z)
    s_z = z;
end
if isempty(ready_land)
    ready_land = false;
end
    
battery_low = false;
for i = 1:UAV_NUM
    if battery_status(i) < battery_threshold
        battery_low = true;
        break;
    end
end
if sim_time_end - timestamp < 1
    tello_stop = true;
else
    tello_stop = false;
end
if battery_low || tello_stop
    if ~ready_land
        ready_land = true;
    end
    z_d_ = z_d_for_land;
    x_d_ = s_x;
    y_d_ = s_y;
else
   ready_land = false;
   s_x = x;
   s_y = y;
   x_d_ = x_d;
   y_d_ = y_d;
   z_d_ = z_d;
end

== matlab function SIMULINK_PID_Tracking_R18b/CMD_car1/CMD5/Subsystem/MATLAB Function ==
  settings: updateMethod=DISCRETE
  data: timestamp input; uavnum input; x_ output; y_ output; z_ output; switch_flag input; stas input; trj_flag input; form_flag input; avo_flag input
function [x_, y_, z_] = fcn(timestamp, uavnum,switch_flag,stas,trj_flag,form_flag,avo_flag)

[x_,y_,z_]=trjcar(timestamp,uavnum,switch_flag,stas,trj_flag,form_flag,avo_flag);

== matlab function SIMULINK_PID_Tracking_R18b/CMD_car1/CMD6/MATLAB Function1 ==
  settings: updateMethod=DISCRETE
  data: x_d input; y_d input; z_d input; timestamp input; x input; y input; z input; battery_status input; sim_time_end input; x_d_ output; battery_threshold input; z_d_for_land input; y_d_ output; z_d_ output; UAV_NUM input
function [x_d_, y_d_, z_d_] = fcn(x_d, y_d, z_d, timestamp, x,y,z,battery_status, sim_time_end,battery_threshold, z_d_for_land, UAV_NUM)
persistent s_x s_y s_z ready_land
if isempty(s_x)
    s_x = x;
end
if isempty(s_y)
    s_y = y;
end
if isempty(s_z)
    s_z = z;
end
if isempty(ready_land)
    ready_land = false;
end
    
battery_low = false;
for i = 1:UAV_NUM
    if battery_status(i) < battery_threshold
        battery_low = true;
        break;
    end
end
if sim_time_end - timestamp < 1
    tello_stop = true;
else
    tello_stop = false;
end
if battery_low || tello_stop
    if ~ready_land
        ready_land = true;
    end
    z_d_ = z_d_for_land;
    x_d_ = s_x;
    y_d_ = s_y;
else
   ready_land = false;
   s_x = x;
   s_y = y;
   x_d_ = x_d;
   y_d_ = y_d;
   z_d_ = z_d;
end

== matlab function SIMULINK_PID_Tracking_R18b/control system_UAV/MATLAB Function ==
  data: u input; y output
function y = fcn(u)
plot(u(1),u(2),"*");
hold on;
y = u;
